simulink model "ctrl_2x2_reves"  (Simulink 7.9)
settings: Solver=FixedStepDiscrete  StartTime=0.0  StopTime=tend  FixedStep=params.th  MaxStep=0.01  RelTol=1e-6  AbsTol=1e-3
values from neighbouring files (symbols this model uses):
  amp_DeltaT1 = -1200    [ctrl_design.m]
  amp_DeltaT2 = +500    (= 500)    [ctrl_design.m]
  delta_t1 = 150    [ctrl_design.m]
  delta_t2 = 300    [ctrl_design.m]
  Gc_pot_d = c2d(Gc_pot,params.th,'tustin')    [ctrl_design.m]
  Gc_vel_d = c2d(Gc_vel,params.th,'tustin')    [ctrl_design.m]
undefined symbols (not defined in the file or in its folder): params
settings Model: Creator=puri  LastModifiedBy=sgpeltoj
settings CodeAppCC: CustomSymbolStrType=$N$R$M_T
settings GRTTargetCC: CodeReplacementLibrary=None  CPPClassGenCompliant=on

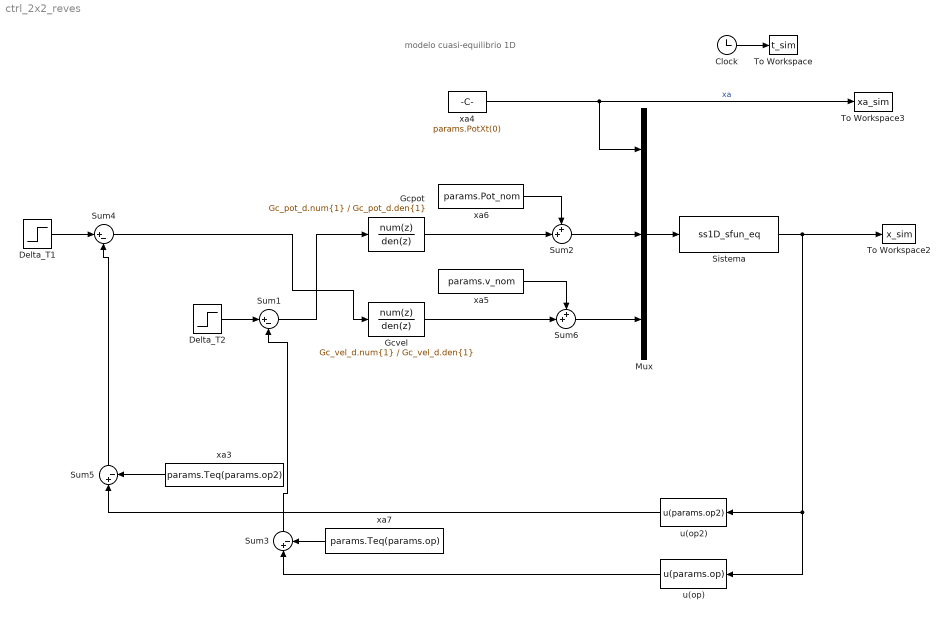
== system ctrl_2x2_reves ==
  note: modelo cuasi-equilibrio 1D
  Clock : Clock
  Delta_T1 : Step  Time=delta_t1  After=amp_DeltaT1  SampleTime=0
  Delta_T2 : Step  Time=delta_t2  After=amp_DeltaT2  SampleTime=0
  Gcpot : DiscreteTransferFcn  Numerator=Gc_pot_d.num{1}  Denominator=Gc_pot_d.den{1}  SampleTime=params.th
  Gcvel : DiscreteTransferFcn  Numerator=Gc_vel_d.num{1}  Denominator=Gc_vel_d.den{1}  SampleTime=params.th
  Mux : Mux  Inputs=3
  Sistema : S-Function  FunctionName=ss1D_sfun_eq  EnableBusSupport=off
      settings: DeleteFcn=shh = get(0,'ShowHiddenHandles');set(0,'ShowHiddenHandles','on');if ~isempty(findobj('type','figure','name','dblcart1 Animation'));close('dblcart1 Animation'); end;set(0,'ShowHiddenHandles',shh);
  Sum{1,3..5} (4 alike) : Sum  Inputs=|+-
  Sum2 : Sum  Inputs=++|
  Sum6 : Sum  Inputs=++|
  To Workspace : ToWorkspace  VariableName=t_sim  SampleTime=-1
  To Workspace2 : ToWorkspace  VariableName=x_sim  SampleTime=-1
  To Workspace3 : ToWorkspace  VariableName=xa_sim  SampleTime=-1
  u(op) : MATLABFcn  MATLABFcn=u(params.op)
  u(op2) : MATLABFcn  MATLABFcn=u(params.op2)
  xa3 : Constant  Value=params.Teq(params.op2)
  xa4 : Constant  Value=params.PotXt(0)
  xa5 : Constant  Value=params.v_nom
  xa6 : Constant  Value=params.Pot_nom
  xa7 : Constant  Value=params.Teq(params.op)
  wires:
  Mux/1 -> Sistema/1
  Sistema/1 -> To Workspace2/1, u(op2)/1, u(op)/1
  xa4/1 -> Mux/1, To Workspace3/1  "xa"
  Clock/1 -> To Workspace/1
  u(op)/1 -> Sum3/1
  xa6/1 -> Sum2/1
  xa5/1 -> Sum6/1
  Delta_T1/1 -> Sum4/1
  Delta_T2/1 -> Sum1/1
  u(op2)/1 -> Sum5/1
  xa3/1 -> Sum5/2
  xa7/1 -> Sum3/2
  Gcpot/1 -> Sum2/2
  Gcvel/1 -> Sum6/2
  Sum2/1 -> Mux/2
  Sum6/1 -> Mux/3
  Sum3/1 -> Sum1/2
  Sum5/1 -> Sum4/2
  Sum1/1 -> Gcpot/1
  Sum4/1 -> Gcvel/1
